simulink model "exercise2_sl"  (R2019b)
settings: Solver=FixedStepAuto  StartTime=0.0  StopTime=0.2  FixedStep=1e-3  RelTol=1e-3  EnableMultiTasking=on
settings Model: ExtModeTrigMode=oneshot  ExtModeArmWhenConnect=off  Creator=lucam  LastModifiedBy=lucam
settings DataIOCC: SaveFormat=Array  SignalLoggingSaveFormat=ModelDataLogs  ReturnWorkspaceOutputs=off
settings OptimizationCC: BlockReduction=off  BooleanDataType=off
settings DebuggingCC: SaveWithParameterizedLinksMsg=none  UnderspecifiedInitializationDetection=Classic  MergeDetectMultiDrivingBlocksExec=none  SignalResolutionControl=TryResolveAllWithWarning  MultiTaskDSMMsg=warning  MultiTaskCondExecSysMsg=none  ArithmeticOperatorsInVariantConditions=warning
settings HardwareCC: TargetUnknown=on
settings ModelReferenceCC: PropagateSignalLabelsOutOfModel=off
settings SFSimCC: SimUseLocalCustomCode=off  CustomCodeUndefinedFunction=UseInterfaceOnly
settings RTWCC: RTWUseLocalCustomCode=off
settings GRTTargetCC: TargetLangStandard=C89/C90 (ANSI)  CombineOutputUpdateFcns=off  GRTInterface=on

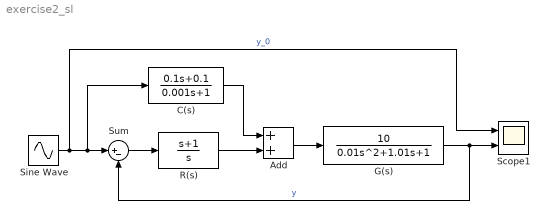
== system exercise2_sl ==
  Add : Sum
  C(s) : TransferFcn  Numerator=[0.1 0.1]  Denominator=[0.001 1]
  G(s) : TransferFcn  Numerator=10  Denominator=[0.01 1.01 1]
  R(s) : TransferFcn  Numerator=[1 1]  Denominator=[1 0]
  Scope1 : Scope  NumInputPorts=2
  Sine Wave : Sin  Frequency=80  SampleTime=0
  Sum : Sum  Inputs=|+-  SaturateOnIntegerOverflow=on  InputSameDT=on  OutDataTypeStr=Inherit: Same as first input
  wires:
  Sum/1 -> R(s)/1
  R(s)/1 -> Add/2
  Add/1 -> G(s)/1
  Sine Wave/1 -> Scope1/1, Sum/1, C(s)/1  "y_0"
  C(s)/1 -> Add/1
  G(s)/1 -> Sum/2, Scope1/2  "y"
